simulink model "Lab_of_P_I__PI_Controllers"  (R2022b)
settings: Solver=VariableStepAuto  StartTime=0.0  StopTime=30  RelTol=1e-3
settings Model: Creator=ahmed  LastModifiedBy=ahmed

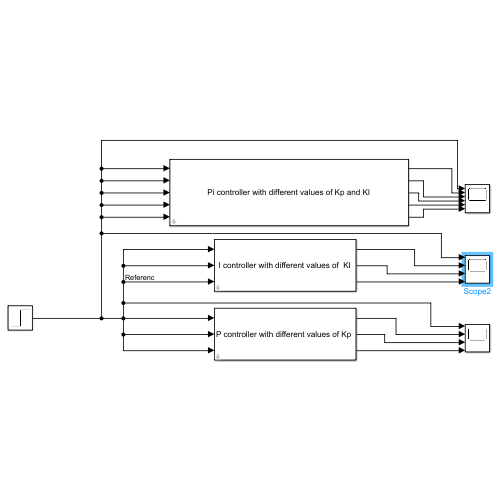
[thumbnail: Simulink's stored preview of the top-level diagram]
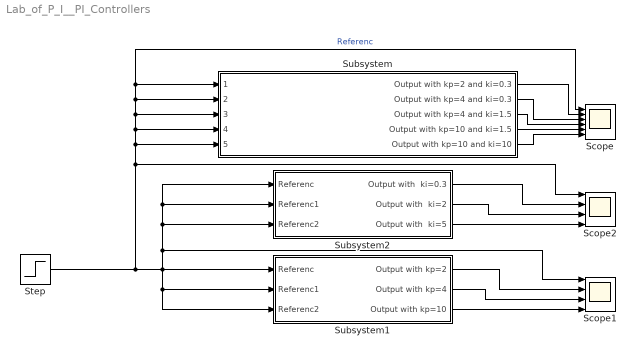
== system Lab_of_P_I__PI_Controllers ==
  Scope : Scope  NumInputPorts=6
  Scope1 : Scope  NumInputPorts=4
  Scope2 : Scope  NumInputPorts=4
  Step : Step  SampleTime=0
  Subsystem : Subsystem
      mask Display: disp('Pi controller with different values of Kp and KI');
  Subsystem1 : Subsystem
      mask Display: disp('P controller with different values of Kp ');
  Subsystem2 : Subsystem
      mask Display: disp('I controller with different values of  KI');
  wires:
  Step/1 -> Subsystem1/2(Referenc1), Subsystem1/3(Referenc2), Scope1/1, Subsystem2/1(Referenc), Subsystem2/2(Referenc1), Subsystem2/3(Referenc2), Subsystem1/1(Referenc), Scope2/1, Scope/1, Subsystem/1(1), Subsystem/2(2), Subsystem/3(3), Subsystem/4(4), Subsystem/5(5)  "Referenc"
  Subsystem/5(Output with kp=10 and ki=10) -> Scope/6
  Subsystem/4(Output with kp=10 and ki=1.5) -> Scope/5
  Subsystem/3(Output with kp=4 and ki=1.5) -> Scope/4
  Subsystem/2(Output with kp=4 and ki=0.3) -> Scope/3
  Subsystem/1(Output with kp=2 and ki=0.3) -> Scope/2
  Subsystem1/1(Output with kp=2) -> Scope1/2
  Subsystem1/2(Output with kp=4) -> Scope1/3
  Subsystem1/3(Output with kp=10) -> Scope1/4
  Subsystem2/2(Output with  ki=2) -> Scope2/3
  Subsystem2/3(Output with  ki=5) -> Scope2/4
  Subsystem2/1(Output with  ki=0.3) -> Scope2/2

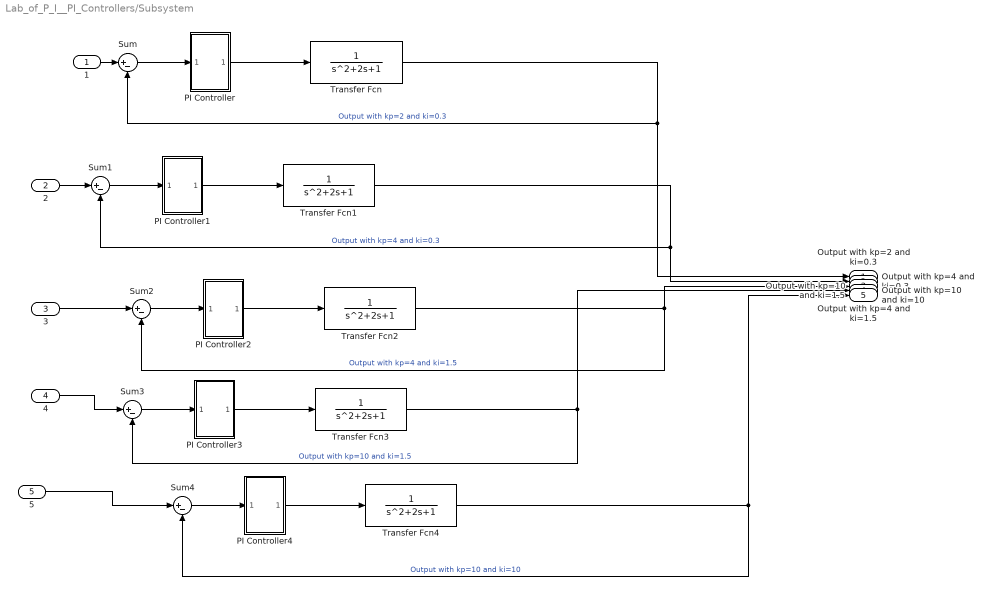
== system Lab_of_P_I__PI_Controllers/Subsystem ==
  1 : Inport
  2 : Inport  Port=2
  3 : Inport  Port=3
  4 : Inport  Port=4
  5 : Inport  Port=5
  PI Controller : Subsystem
  PI Controller1 : Subsystem
  PI Controller2 : Subsystem
  PI Controller3 : Subsystem
  PI Controller4 : Subsystem
  Sum{,1..4} (5 alike) : Sum  Inputs=|+-
  Transfer Fcn{,1..4} (5 alike) : TransferFcn
  Output with kp=2 and ki=0.3 : Outport
  Output with kp=4 and ki=0.3 : Outport  Port=2
  Output with kp=4 and ki=1.5 : Outport  Port=3
  Output with kp=10 and ki=1.5 : Outport  Port=4
  Output with kp=10 and ki=10 : Outport  Port=5
  wires:
  PI Controller2/1(Out1) -> Transfer Fcn2/1
  Transfer Fcn2/1 -> Output with kp=4 and ki=1.5/1, Sum2/2  "Output with kp=4 and ki=1.5"
  Transfer Fcn4/1 -> Output with kp=10 and ki=10/1, Sum4/2  "Output with kp=10 and ki=10"
  Transfer Fcn1/1 -> Output with kp=4 and ki=0.3/1, Sum1/2  "Output with kp=4 and ki=0.3"
  Transfer Fcn3/1 -> Output with kp=10 and ki=1.5/1, Sum3/2  "Output with kp=10 and ki=1.5"
  5/1 -> Sum4/1
  Sum1/1 -> PI Controller1/1(In1)
  PI Controller1/1(Out1) -> Transfer Fcn1/1
  Sum2/1 -> PI Controller2/1(In1)
  Sum4/1 -> PI Controller4/1(In1)
  PI Controller4/1(Out1) -> Transfer Fcn4/1
  Sum/1 -> PI Controller/1(In1)
  PI Controller3/1(Out1) -> Transfer Fcn3/1
  Sum3/1 -> PI Controller3/1(In1)
  Transfer Fcn/1 -> Output with kp=2 and ki=0.3/1, Sum/2  "Output with kp=2 and ki=0.3"
  PI Controller/1(Out1) -> Transfer Fcn/1
  2/1 -> Sum1/1
  3/1 -> Sum2/1
  4/1 -> Sum3/1
  1/1 -> Sum/1

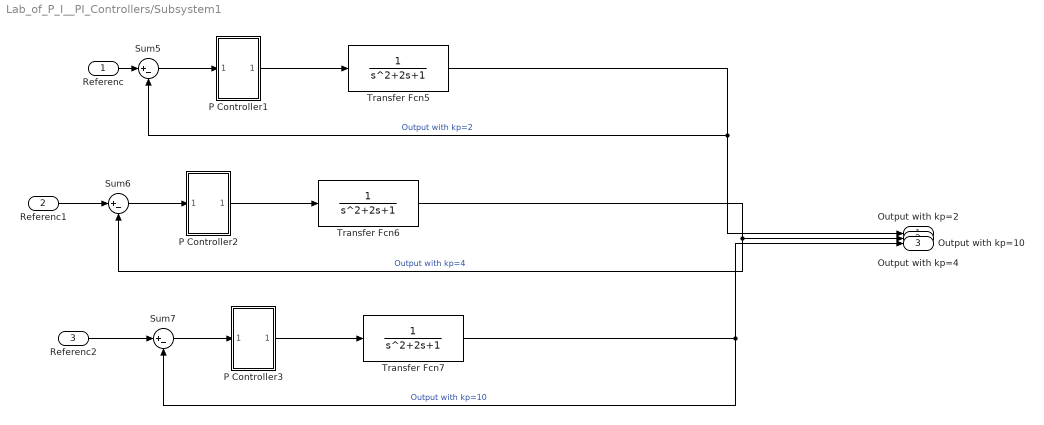
== system Lab_of_P_I__PI_Controllers/Subsystem1 ==
  Referenc : Inport
  Referenc1 : Inport  Port=2
  Referenc2 : Inport  Port=3
  P Controller1 : Subsystem
  P Controller2 : Subsystem
  P Controller3 : Subsystem
  Sum5 : Sum  Inputs=|+-
  Sum6 : Sum  Inputs=|+-
  Sum7 : Sum  Inputs=|+-
  Transfer Fcn5 : TransferFcn
  Transfer Fcn6 : TransferFcn
  Transfer Fcn7 : TransferFcn
  Output with kp=2 : Outport
  Output with kp=4 : Outport  Port=2
  Output with kp=10 : Outport  Port=3
  wires:
  P Controller2/1(Out1) -> Transfer Fcn6/1
  P Controller3/1(Out1) -> Transfer Fcn7/1
  Sum6/1 -> P Controller2/1(In1)
  Transfer Fcn6/1 -> Output with kp=4/1, Sum6/2  "Output with kp=4"
  Sum5/1 -> P Controller1/1(In1)
  P Controller1/1(Out1) -> Transfer Fcn5/1
  Transfer Fcn5/1 -> Output with kp=2/1, Sum5/2  "Output with kp=2"
  Transfer Fcn7/1 -> Output with kp=10/1, Sum7/2  "Output with kp=10"
  Sum7/1 -> P Controller3/1(In1)
  Referenc1/1 -> Sum6/1
  Referenc/1 -> Sum5/1
  Referenc2/1 -> Sum7/1

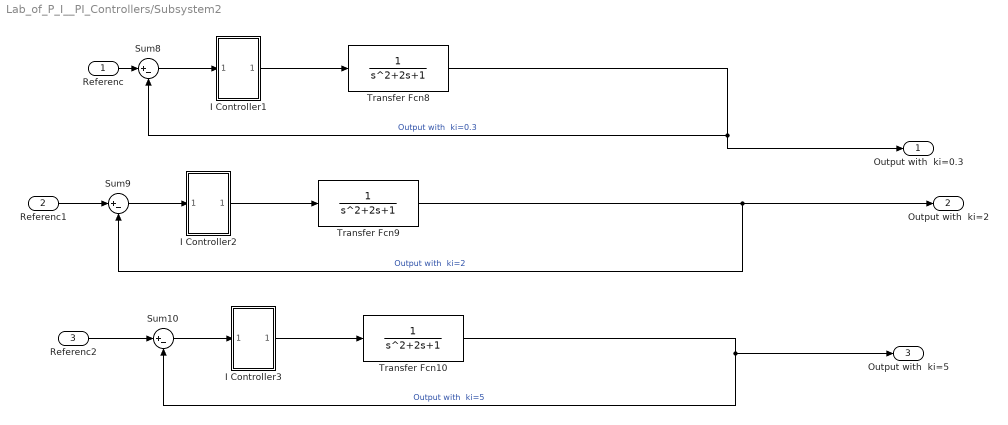
== system Lab_of_P_I__PI_Controllers/Subsystem2 ==
  Referenc : Inport
  Referenc1 : Inport  Port=2
  Referenc2 : Inport  Port=3
  I Controller1 : Subsystem
  I Controller2 : Subsystem
  I Controller3 : Subsystem
  Sum10 : Sum  Inputs=|+-
  Sum8 : Sum  Inputs=|+-
  Sum9 : Sum  Inputs=|+-
  Transfer Fcn10 : TransferFcn
  Transfer Fcn8 : TransferFcn
  Transfer Fcn9 : TransferFcn
  Output with  ki=0.3 : Outport
  Output with  ki=2 : Outport  Port=2
  Output with  ki=5 : Outport  Port=3
  wires:
  I Controller1/1(Out1) -> Transfer Fcn8/1
  Referenc2/1 -> Sum10/1
  Transfer Fcn10/1 -> Output with  ki=5/1, Sum10/2  "Output with  ki=5"
  I Controller3/1(Out1) -> Transfer Fcn10/1
  Transfer Fcn9/1 -> Sum9/2, Output with  ki=2/1  "Output with  ki=2"
  Sum8/1 -> I Controller1/1(In1)
  Sum10/1 -> I Controller3/1(In1)
  Sum9/1 -> I Controller2/1(In1)
  I Controller2/1(Out1) -> Transfer Fcn9/1
  Transfer Fcn8/1 -> Output with  ki=0.3/1, Sum8/2  "Output with  ki=0.3"
  Referenc1/1 -> Sum9/1
  Referenc/1 -> Sum8/1

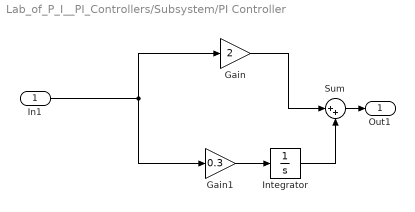
== system Lab_of_P_I__PI_Controllers/Subsystem/PI Controller ==
  In1 : Inport
  Gain : Gain  Gain=2
  Gain1 : Gain  Gain=0.3
  Integrator : Integrator
  Sum : Sum  Inputs=|++
  Out1 : Outport
  wires:
  In1/1 -> Gain/1, Gain1/1
  Gain/1 -> Sum/1
  Integrator/1 -> Sum/2
  Gain1/1 -> Integrator/1
  Sum/1 -> Out1/1

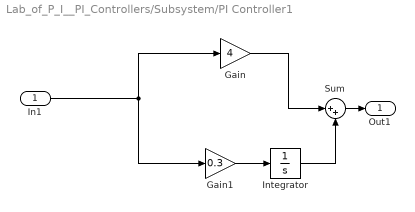
== system Lab_of_P_I__PI_Controllers/Subsystem/PI Controller1 ==
  In1 : Inport
  Gain : Gain  Gain=4
  Gain1 : Gain  Gain=0.3
  Integrator : Integrator
  Sum : Sum  Inputs=|++
  Out1 : Outport
  wires:
  Sum/1 -> Out1/1
  Gain1/1 -> Integrator/1
  Integrator/1 -> Sum/2
  Gain/1 -> Sum/1
  In1/1 -> Gain1/1, Gain/1

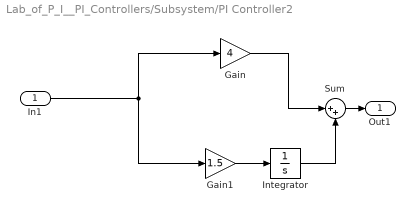
== system Lab_of_P_I__PI_Controllers/Subsystem/PI Controller2 ==
  In1 : Inport
  Gain : Gain  Gain=4
  Gain1 : Gain  Gain=1.5
  Integrator : Integrator
  Sum : Sum  Inputs=|++
  Out1 : Outport
  wires:
  In1/1 -> Gain/1, Gain1/1
  Gain/1 -> Sum/1
  Integrator/1 -> Sum/2
  Gain1/1 -> Integrator/1
  Sum/1 -> Out1/1

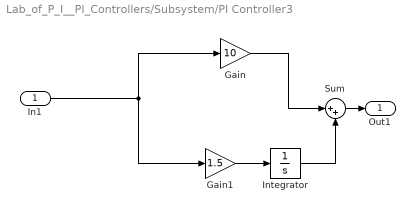
== system Lab_of_P_I__PI_Controllers/Subsystem/PI Controller3 ==
  In1 : Inport
  Gain : Gain  Gain=10
  Gain1 : Gain  Gain=1.5
  Integrator : Integrator
  Sum : Sum  Inputs=|++
  Out1 : Outport
  wires:
  Sum/1 -> Out1/1
  Gain1/1 -> Integrator/1
  Integrator/1 -> Sum/2
  Gain/1 -> Sum/1
  In1/1 -> Gain1/1, Gain/1

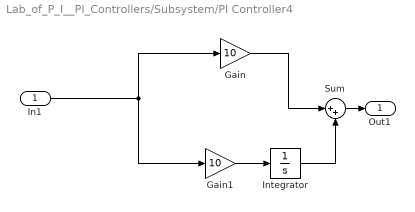
== system Lab_of_P_I__PI_Controllers/Subsystem/PI Controller4 ==
  In1 : Inport
  Gain : Gain  Gain=10
  Gain1 : Gain  Gain=10
  Integrator : Integrator
  Sum : Sum  Inputs=|++
  Out1 : Outport
  wires:
  In1/1 -> Gain/1, Gain1/1
  Gain/1 -> Sum/1
  Integrator/1 -> Sum/2
  Gain1/1 -> Integrator/1
  Sum/1 -> Out1/1

== system Lab_of_P_I__PI_Controllers/Subsystem1/P Controller1 ==
  In1 : Inport
  Gain : Gain  Gain=2
  Out1 : Outport
  wires:
  Gain/1 -> Out1/1
  In1/1 -> Gain/1

== system Lab_of_P_I__PI_Controllers/Subsystem1/P Controller2 ==
  In1 : Inport
  Gain : Gain  Gain=4
  Out1 : Outport
  wires:
  In1/1 -> Gain/1
  Gain/1 -> Out1/1

== system Lab_of_P_I__PI_Controllers/Subsystem1/P Controller3 ==
  In1 : Inport
  Gain : Gain  Gain=10
  Out1 : Outport
  wires:
  Gain/1 -> Out1/1
  In1/1 -> Gain/1

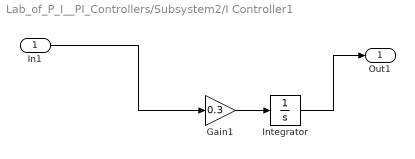
== system Lab_of_P_I__PI_Controllers/Subsystem2/I Controller1 ==
  In1 : Inport
  Gain1 : Gain  Gain=0.3
  Integrator : Integrator
  Out1 : Outport
  wires:
  Integrator/1 -> Out1/1
  Gain1/1 -> Integrator/1
  In1/1 -> Gain1/1

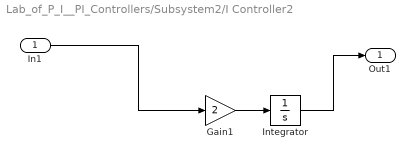
== system Lab_of_P_I__PI_Controllers/Subsystem2/I Controller2 ==
  In1 : Inport
  Gain1 : Gain  Gain=2
  Integrator : Integrator
  Out1 : Outport
  wires:
  In1/1 -> Gain1/1
  Gain1/1 -> Integrator/1
  Integrator/1 -> Out1/1

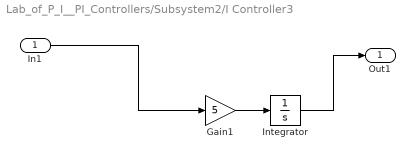
== system Lab_of_P_I__PI_Controllers/Subsystem2/I Controller3 ==
  In1 : Inport
  Gain1 : Gain  Gain=5
  Integrator : Integrator
  Out1 : Outport
  wires:
  Integrator/1 -> Out1/1
  Gain1/1 -> Integrator/1
  In1/1 -> Gain1/1
